simulink model "complexifft4"  (R2021b)
settings: Solver=VariableStepAuto  StartTime=0.0  StopTime=10.0  RelTol=1e-3
libraries: hdlBasic x17, xbsIndex_r4 x1
settings Model: Creator=Apoorv  LastModifiedBy=Apoorv

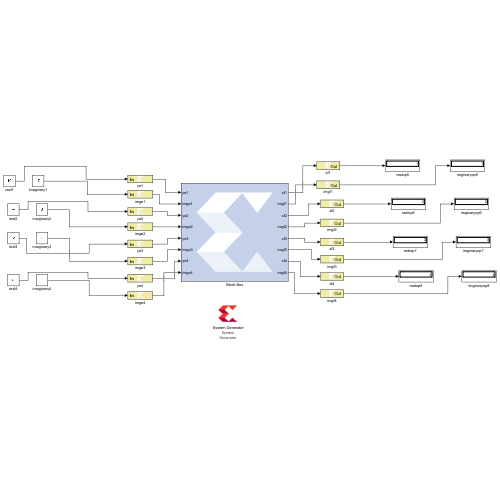
[thumbnail: Simulink's stored preview of the top-level diagram]
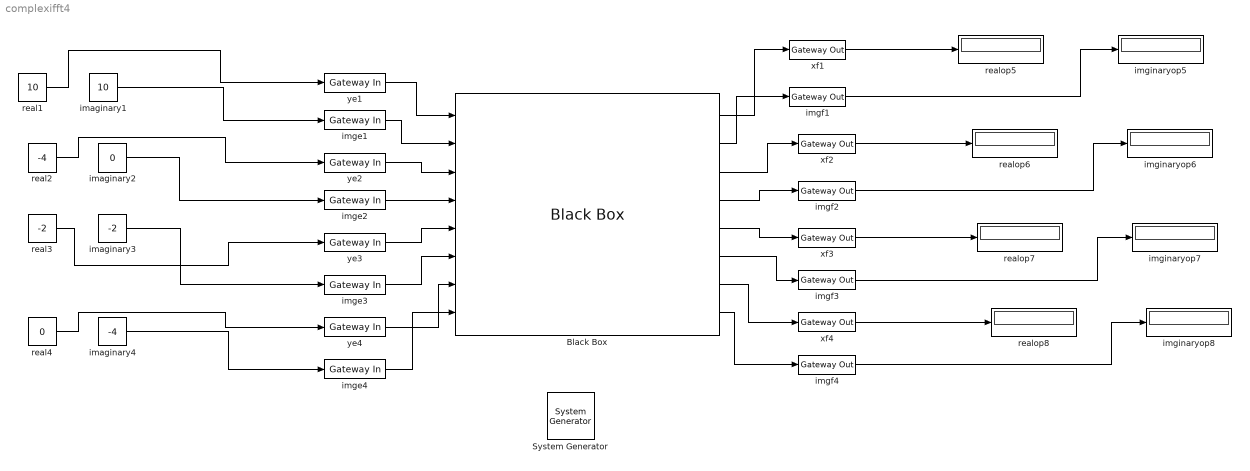
== system complexifft4 ==
  " System Generator" : xbsIndex_r4/ System Generator  Tag=genX  xilinxfamily=kintex7  part=xc7k160t  speed=-1  package=fbg484  synthesis_tool=Vivado  clock_wrapper=Clock Enables  directory=./netlist  proj_type=Vivado  Synth_file=Vivado Synthesis Defaults  Impl_file=Vivado Implementation Defaults  testbench=off  simulink_period=1  sysclk_period=10  dcm_input_clock_period=10  incr_netlist=off  trim_vbits=Everywhere in SubSystem  dbl_ovrd=According to Block Masks  core_generation=According to Block Masks  run_coregen=off  deprecated_control=off  eval_field=0  block_type=sysgen
  Black Box : hdlBasic/Black Box  init_code=compifft4_config  sim_method=Vivado Simulator  verbose=off  XmcBlockStatus=1  maskContainerNames=group1  block_type=blackbox2  block_config=sysgen:black_box_config
  imaginary1 : Constant  Value=10
  imaginary2 : Constant  Value=0
  imaginary3 : Constant  Value=-2
  imaginary4 : Constant  Value=-4
  imge{1..4} (4 alike) : hdlBasic/Gateway In  gui_display_data_type=Fixed-point  arith_type=Signed (2's comp)  n_bits=8  bin_pt=0  preci_type=Single  exp_width=8  frac_width=24  rows=1  columns=1  quantization="Round  (unbiased: +/- Inf)"  overflow=Saturate  period=1  UseAsADC=off  ADCChannel='1'  interface=None  automatic_assignment=on  address_offset=hex2dec('00')  intf_name=''  intf_description=''  default_value=0  timing_constraint=None  locs_specified=off  LOCs={}  io_standard={}  inherit_from_input=off  hdl_port=on  XmcBlockStatus=1  maskContainerNames=group4  block_type=gatewayin  block_config=sysgen:gateway_in_config  block_width_w=590  block_height_w=620  block_width=640  block_height=850
  imgf{1..4} (4 alike) : hdlBasic/Gateway Out  inherit_from_input=on  hdl_port=off  rows=1  columns=1  UseAsDAC=off  DACChannel='1'  interface=None  automatic_assignment=on  address_offset=hex2dec('00')  intf_name=''  intf_description=''  timing_constraint=None  locs_specified=off  LOCs={}  io_standard={}  XmcBlockStatus=1  maskContainerNames=group4  block_type=gatewayout  block_config=sysgen:gateway_out_config  block_width_w=590  block_height_w=620  block_width=620  block_height=750
  imginaryop{5..8} (4 alike) : Display
      settings: Format=decimal (Stored Integer)
  real1 : Constant  Value=10
  real2 : Constant  Value=-4
  real3 : Constant  Value=-2
  real4 : Constant  Value=0
  realop{5..8} (4 alike) : Display
      settings: Format=decimal (Stored Integer)
  xf{1..4} (4 alike) : hdlBasic/Gateway Out  inherit_from_input=on  hdl_port=off  rows=1  columns=1  UseAsDAC=off  DACChannel='1'  interface=None  automatic_assignment=on  address_offset=hex2dec('00')  intf_name=''  intf_description=''  timing_constraint=None  locs_specified=off  LOCs={}  io_standard={}  XmcBlockStatus=1  maskContainerNames=group4  block_type=gatewayout  block_config=sysgen:gateway_out_config  block_width_w=590  block_height_w=620  block_width=620  block_height=750
  ye{1..4} (4 alike) : hdlBasic/Gateway In  gui_display_data_type=Fixed-point  arith_type=Signed (2's comp)  n_bits=8  bin_pt=0  preci_type=Single  exp_width=8  frac_width=24  rows=1  columns=1  quantization="Round  (unbiased: +/- Inf)"  overflow=Saturate  period=1  UseAsADC=off  ADCChannel='1'  interface=None  automatic_assignment=on  address_offset=hex2dec('00')  intf_name=''  intf_description=''  default_value=0  timing_constraint=None  locs_specified=off  LOCs={}  io_standard={}  inherit_from_input=off  hdl_port=on  XmcBlockStatus=1  maskContainerNames=group4  block_type=gatewayin  block_config=sysgen:gateway_in_config  block_width_w=590  block_height_w=620  block_width=640  block_height=850
  wires:
  real4/1 -> ye4/1
  imaginary3/1 -> imge3/1
  imaginary4/1 -> imge4/1
  imaginary2/1 -> imge2/1
  real3/1 -> ye3/1
  real2/1 -> ye2/1
  real1/1 -> ye1/1
  imaginary1/1 -> imge1/1
  ye1/1 -> Black Box/1
  imge1/1 -> Black Box/2
  ye2/1 -> Black Box/3
  imge2/1 -> Black Box/4
  ye3/1 -> Black Box/5
  imge3/1 -> Black Box/6
  ye4/1 -> Black Box/7
  imge4/1 -> Black Box/8
  imgf3/1 -> imginaryop7/1
  imgf2/1 -> imginaryop6/1
  xf4/1 -> realop8/1
  xf3/1 -> realop7/1
  imgf4/1 -> imginaryop8/1
  xf1/1 -> realop5/1
  imgf1/1 -> imginaryop5/1
  xf2/1 -> realop6/1
  Black Box/1 -> xf1/1
  Black Box/2 -> imgf1/1
  Black Box/3 -> xf2/1
  Black Box/4 -> imgf2/1
  Black Box/5 -> xf3/1
  Black Box/6 -> imgf3/1
  Black Box/7 -> xf4/1
  Black Box/8 -> imgf4/1
